simulink model "RWLNN_2m__fcn"  (R2015b)
settings: Solver=ode1  StartTime=0.0  StopTime=t_sim  FixedStep=t_prob  RelTol=1e-3
values from neighbouring files (symbols this model uses):
  ksi = 1    [RWLNN_weights (2).mat]
  lr = 0.01    [RWLNN_weights (2).mat]
  lra = 0.001    [RWLNN_weights (2).mat]
  lrb = 0.001    [RWLNN_weights (2).mat]
  lrin = 0.001    [RWLNN_weights (2).mat]
  T1 = 0.203    [RWLNN_weights (2).mat]
  T2 = 0.203    [RWLNN_weights (2).mat]
  t_prob = 0.0001    [RWLNN_weights (2).mat]
  Tc = 0.0012    [RWLNN_weights (2).mat]
  w0 = 40    [RWLNN_weights (2).mat]
  w_init = [0.41  0  0.42; 0  0  -0.04]    [RWLNN_weights (2).mat]
  w_out_init = [-5 0 5]    [RWLNN_weights (2).mat]
undefined symbols (not defined in the file or in its folder): Lz, sysd, sysd1
libraries: neural x3, simulink x2
(part 2 of 2)

== matlab function RWLNN_2m__fcn/MATLAB Function1 ==
  data: em input; y_out output; lr input; in1 input; in2 input
function y_out    = rwlnn(em, lr, in1,in2)

persistent a b w w_out l1_in l1_min1 l1_out l2_in l2_out l3_in l3_out ...
    l3_r_in l3_r_out l4_r_in l4_r_out l4_in l4_out ...
    delta_w_out delta_3 delta_2 delta_1 delta_a delta_b delta_w lra lrb lr_w w_rec

%% Initialize

lra = 0.001;
lrb = 0.001;
lr_w = 0.001;
if isempty(w)
    w = [0.41 0 0.42; 0 0 -0.04];
%     w = randn(2,3)./10; 
end

if isempty(a)
    a = [-0.34 0.5 0.36; -0.26 0.4 0.26];
%     a = rand(2,3); 
end

if isempty(b)
    b = [0.56 1.02 0.54; 1.12 1 1.13];
%     b = randn(2,3);
end

if isempty(w_out)
    w_out = [-5 0 5];
end

if isempty(l1_in)
    l1_in = zeros(2,3);
end

if isempty(l1_min1)
    l1_min1 = zeros(2,3);
end

if isempty(l1_out)
    l1_out = zeros(2,3);
end

if isempty(l2_in)
    l2_in = zeros(2,3);
end

if isempty(l2_out)
    l2_out = zeros(2,3);
end

if isempty(l3_in)
    l3_in = zeros(1,3);
end

if isempty(l3_out)
    l3_out = zeros(1,3);
end

if isempty(l3_r_in)
    l3_r_in = zeros(1,3);
end

if isempty(l3_r_out)
    l3_r_out = zeros(1,3);
end

if isempty(l4_in)
    l4_in = zeros(1,3);
end

if isempty(l4_out)
    l4_out = zeros(1,1);
end

if isempty(l4_r_in)
    l4_r_in = zeros(1,1);
end

if isempty(l4_r_out)
    l4_r_out = zeros(1,1);
end

if isempty(delta_w_out)
    delta_w_out = zeros(1,3);
end

if isempty(delta_3)
    delta_3 = zeros(1,3);
end

if isempty(delta_2)
    delta_2 = zeros(2,3);
end

if isempty(delta_1)
    delta_1 = zeros(2,3);
end

if isempty(delta_w)
    delta_w = zeros(2,3);
end

if isempty(delta_a)
    delta_a = zeros(2,3);
end

if isempty(delta_b)
    delta_b = zeros(2,3);
end

if isempty(w_rec)
    w_rec = rand./10;
end

%% Forward Pass

y_out = 0;

l1_min1(1,:) = w(1,:) .* l1_in(1,:);    % Previous samples for x1
l1_min1(2,:) = w(2,:) .* l1_in(2,:);    %                      x2

l1_in(1,:)   = in1 + l1_min1(1,:);      % Present values x1
l1_in(2,:)   = in2 + l1_min1(2,:);      % 

l1_out       = l1_in;                   % L1 - linear neuron

l2_in        = (l1_out - a)./b;         % L2 input
l2_out       = cos(0.25 * l2_in) .* exp(-(l2_in) .^ 2); % L2 output - mother wavelet

l3_r_out     = 1 ./ (1 + exp(-l3_r_in));% Previous recurrent L3 output

l4_r_out     = exp(-(l4_r_in)^2);       % Previous recurrent L4 output

for i = 1:3         % For all wavelets (3) 
    
    l3_in(i) = l2_out(1, i) * l2_out(2, i) * l3_r_out(i)  * l4_r_out;
    
end

l3_out   = l3_in;                       % L3 output - product of L2 and recurrences
   
l3_r_in  = l3_out;                      % Present L3 recurrent input

l4_r_in  = w_rec * y_out;               % Present L4 recurrent input

l4_in    = l3_out .* w_out;             % Present L4 input

l4_out   = sum(l4_in);                  % Present L4 output - sum of L3 outputs times weights

y_out    = l4_out;                      % Output

%% Backpropagation

delta_w_out = lr * em * l3_out;
delta_3     = em * w_out;
w_out       = w_out + delta_w_out;
w_rec       = w_rec + (lr * em * y_out);

for i = 1:2
    for j = 1:3
        delta_2(i,j) = delta_3(j) * l4_r_out * l3_r_out(j) * l2_out(i,j);
    end
end

delta_a = lra .* delta_2 .* (2 .* l2_in .* exp(- (l2_in).^2) .* cos(0.25 .* l2_in) + ...
    0.25 .* exp(-(l2_in).^2) .* sin(0.25 .* l2_in)) .* (1./b);

delta_b = lrb .* delta_2 .* (2 .* l2_in .* exp(- (l2_in).^2) .* cos(0.25 .* l2_in) + ...
    0.25 .* exp(-(l2_in).^2) .* sin(0.25 .* l2_in)) .* l2_in .* (1./b);

a = a + delta_a;
b = b + delta_b;

delta_1 = delta_2 .* (2 .* ((l1_out - a)./b) .* exp(- ((l1_out - a)./b).^2) .* ...
    cos(0.25 .* ((l1_out - a)./b)) + 0.25 .* exp(- ((l1_out - a)./b).^2) .* ...
    sin(0.25 .* ((l1_out - a)./b)) ) .* (-1)./b;

delta_w = lr_w .* delta_1 .* l1_min1;
w = w + delta_w;
end

== matlab function RWLNN_2m__fcn/Subsystem1/MATLAB Function ==
  data: in input; pred output; grad output
function [pred, grad] = fcn(in)

persistent w lr

if(isempty(w))
    w = rand(3,1)./10;
end

if(isempty(lr))
    lr = 0.1;
end

pred = sum(in .* w);

grad = (pred -  in(1)) .* in;

w = w - (lr * grad);

end

== matlab function RWLNN_2m__fcn/Subsystem2/MATLAB Function ==
  data: in input; in2 input; estym output; grad input
function estym = fcn(in, in2, grad)

persistent w lr

if(isempty(w))
    w = rand(3,2)./10;
end

if(isempty(lr))
    lr = 0.01;
end

estym = sum(in .* w(:,1) + in2 .* w(:,2));

w = w - (lr * grad);

end

== matlab function RWLNN_2m__fcn/Subsystem6/MATLAB Function ==
  data: in input; pred output; grad output
function [pred, grad] = fcn(in)

persistent w lr

if(isempty(w))
    w = rand(3,1)./10;
end

if(isempty(lr))
    lr = 0.1;
end

pred = sum(in .* w);

grad = (pred -  in(1)) .* in;

w = w - (lr * grad);

end
